simulink model "gm_sla_VHT_HDL1080p_fil_org"  (R2015a)
settings: Solver=FixedStepDiscrete  SolverMode=SingleTasking  StartTime=0.0  StopTime=2200*1125*100  FixedStep=1  RelTol=1e-3
PreLoadFcn:
  | H = fspecial('unsharp')
undefined symbols (not defined in the file): gray
libraries: simulink x6, visionsinks x3, visionhdlio x2, visionhdlconversions x1, visionhdlfilter x1, fillib x1, visionconversions x1, visiongeotforms x1, dspvision x1
settings Model: SimulationMode=accelerator  CovSFcnEnable=off  Creator=yutengz  LastModifiedBy=amatsumo
settings OptimizationCC: BlockReduction=off  BooleanDataType=off  ConditionallyExecuteInputs=off  InlineParams=on
settings DebuggingCC: AlgebraicLoopMsg=error  SaveWithParameterizedLinksMsg=none  UnderspecifiedInitializationDetection=Classic  MergeDetectMultiDrivingBlocksExec=none  SignalResolutionControl=TryResolveAllWithWarning  InheritedTsInSrcMsg=none
settings HardwareCC: ProdHWDeviceType=ASIC/FPGA->ASIC/FPGA  TargetUnknown=on  ProdEqTarget=off

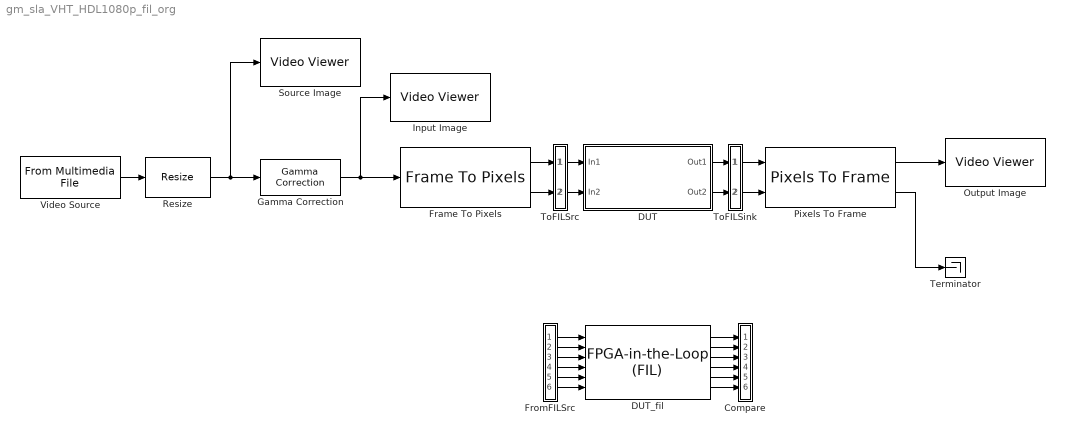
== system gm_sla_VHT_HDL1080p_fil_org ==
  Compare : Subsystem
      mask Display: disp('')
  DUT : Subsystem
  DUT_fil : fillib/FPGA-in-the-Loop (FIL)  ForceInterfaceUpdate=0.90579
  Frame To Pixels : visionhdlio/Frame To Pixels  NumComponents=1  VideoFormat=1080p  ActivePixelsPerLine=32  ActiveVideoLines=18  TotalPixelsPerLine=42  TotalVideoLines=28  StartingActiveLine=6  FrontPorch=5  SampleTime=0
  FromFILSrc : Subsystem
      mask Display: disp('')
  Gamma Correction : visionconversions/Gamma Correction  operation=De-gamma  gamma=2.2  linearSegment=on  breakPoint=0.018
  Input Image : visionsinks/Video Viewer  inputType=Obsolete7b  imagePorts=One multidimensional signal  useColorMap=off  colormapValue=gray(256)  specRange=off  minInputVal=0  maxInputVal=255  FigPos=[366 381 334 275]  AxisZoom=on  trueSizedOnce=off  OpenAtMdlStart=on  DefaultConfigurationName=vipscopes.VideoViewerScopeCfg
  Output Image : visionsinks/Video Viewer  inputType=Obsolete7b  imagePorts=One multidimensional signal  useColorMap=off  colormapValue=gray(256)  specRange=off  minInputVal=0  maxInputVal=255  FigPos=[709 384 334 275]  AxisZoom=on  trueSizedOnce=off  OpenAtMdlStart=on  DefaultConfigurationName=vipscopes.VideoViewerScopeCfg
  Pixels To Frame : visionhdlio/Pixels To Frame  NumComponents=1  VideoFormat=1080p  ActivePixelsPerLine=32  ActiveVideoLines=18  TotalPixelsPerLine=42  TotalVideoLines=28
  Resize : visiongeotforms/Resize  specify=Number of output rows and columns  rfactor=[200 150]  outCols=25  outRows=25  outRowsCols=[1080 1920]  interp_method=Bilinear  antialias=on  useROI=off  roiFlag=off  prodOutputMode=Binary point scaling  prodOutputWordLength=32  prodOutputFracLength=10  roundingMode=Nearest  overflowMode=on
  Source Image : visionsinks/Video Viewer  inputType=Obsolete7b  imagePorts=One multidimensional signal  useColorMap=off  colormapValue=gray(256)  specRange=off  minInputVal=0  maxInputVal=255  FigPos=[21 379 334 275]  AxisZoom=on  trueSizedOnce=off  OpenAtMdlStart=on  DefaultConfigurationName=vipscopes.VideoViewerScopeCfg
  Terminator : Terminator
  ToFILSink : Subsystem
      mask Display: disp('')
  ToFILSrc : Subsystem
      mask Display: disp('')
  Video Source : dspvision/From Multimedia File  inputFilename=rhinos.avi  loop=on  numPlays=inf  outputStreams=Video only  videoDataType=uint8  audioDataType=int16  inheritSampleTime=off  userDefinedSampleTime="1125*2200  %402*324"  noAudioOutput=off  isIntensityVideo=off  fourcc=Intensity  colorVideoFormat=One multidimensional signal  outputEOF=off  dataOrg=Column-major  audioFrameSize=1024  computeAudioFrameSize=off  outSamplingMode=Sample based
  wires:
  Video Source/1 -> Resize/1
  Pixels To Frame/1 -> Output Image/1
  Pixels To Frame/2 -> Terminator/1
  Gamma Correction/1 -> Input Image/1, Frame To Pixels/1
  Resize/1 -> Source Image/1, Gamma Correction/1
  ToFILSrc/1(out1) -> DUT/1(In1)
  ToFILSrc/2(out2) -> DUT/2(In2)
  DUT/1(Out1) -> ToFILSink/1(in1)
  DUT/2(Out2) -> ToFILSink/2(in2)
  Frame To Pixels/1 -> ToFILSrc/1(in1)
  Frame To Pixels/2 -> ToFILSrc/2(in2)
  ToFILSink/1(out1) -> Pixels To Frame/1
  ToFILSink/2(out2) -> Pixels To Frame/2
  FromFILSrc/1(out1) -> DUT_fil/1
  FromFILSrc/2(out2) -> DUT_fil/2
  FromFILSrc/3(out3) -> DUT_fil/3
  FromFILSrc/4(out4) -> DUT_fil/4
  FromFILSrc/5(out5) -> DUT_fil/5
  FromFILSrc/6(out6) -> DUT_fil/6
  DUT_fil/1 -> Compare/1(in1)
  DUT_fil/2 -> Compare/2(in2)
  DUT_fil/3 -> Compare/3(in3)
  DUT_fil/4 -> Compare/4(in4)
  DUT_fil/5 -> Compare/5(in5)
  DUT_fil/6 -> Compare/6(in6)

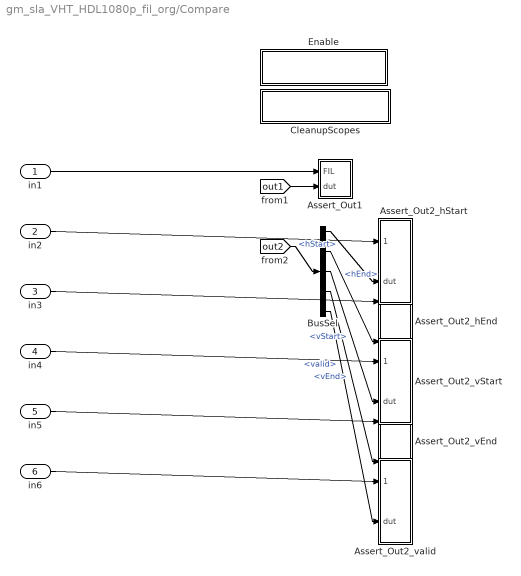
== system gm_sla_VHT_HDL1080p_fil_org/Compare ==
  in1 : Inport
  in2 : Inport  Port=2
  in3 : Inport  Port=3
  in4 : Inport  Port=4
  in5 : Inport  Port=5
  in6 : Inport  Port=6
  Assert_Out1 : Subsystem
  Assert_Out2_hEnd : Subsystem
  Assert_Out2_hStart : Subsystem
  Assert_Out2_vEnd : Subsystem
  Assert_Out2_vStart : Subsystem
  Assert_Out2_valid : Subsystem
  BusSel : BusSelector  OutputSignals=hStart,hEnd,vStart,vEnd,valid
  CleanupScopes : Subsystem
      settings: OpenFcn=|
      | blkName = gcb;
      | idx = regexp(blkName, '/CleanupScopes$', 'once');
      | blkParent = blkName(1:idx-1);
      | blks=find_system(blkParent, 'blocktype', 'Scope');
      | e = get_param(blks{1}, 'Open');
      | if strcmp(e, 'on'), f= 'off'; else f = 'on'; end
      | for ii=1:length(blks), set_param(blks{ii}, 'Open', f); end; drawnow;
      mask Display: disp(['Double click to\n turn on/off all scopes'])
  Enable : Subsystem
      settings: OpenFcn=|
      | blkName = gcb;
      | idx = regexp(blkName, '/Enable$', 'once');
      | blkParent = blkName(1:idx-1);
      | blks=find_system(blkParent, 'blocktype', 'Assertion');
      | e = get_param(blks{1}, 'Enabled');
      | if strcmp(e, 'on'), f= 'off';, else, f = 'on';, end
      | for ii=1:length(blks), set_param(blks{ii}, 'Enabled', f);, end
      | dispMsg = sprintf('disp([''Double click to turn %s \\n all Assertions''])', upper(e));
      | set_param(gcb, 'MaskDisplay', dispMsg);
      mask Display: disp(['Double click to turn OFF \n all Assertions'])
  wires:
  [out2] -> BusSel/1
  in1/1 -> Assert_Out1/1(FIL)
  [out1] -> Assert_Out1/2(dut)
  in2/1 -> Assert_Out2_hStart/1(cosim)
  BusSel/1 -> Assert_Out2_hStart/2(dut)  "<hStart>"
  in3/1 -> Assert_Out2_hEnd/1(cosim)
  BusSel/2 -> Assert_Out2_hEnd/2(dut)  "<hEnd>"
  in4/1 -> Assert_Out2_vStart/1(cosim)
  BusSel/3 -> Assert_Out2_vStart/2(dut)  "<vStart>"
  in5/1 -> Assert_Out2_vEnd/1(cosim)
  BusSel/4 -> Assert_Out2_vEnd/2(dut)  "<vEnd>"
  in6/1 -> Assert_Out2_valid/1(cosim)
  BusSel/5 -> Assert_Out2_valid/2(dut)  "<valid>"

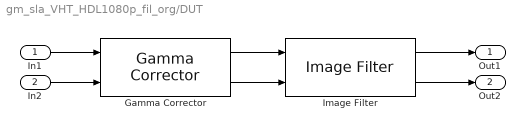
== system gm_sla_VHT_HDL1080p_fil_org/DUT ==
  In1 : Inport
  In2 : Inport  Port=2
  Gamma Corrector : visionhdlconversions/Gamma Corrector  Correction=Gamma  Gamma=2.2  LinearSegment=on  BreakPoint=0.018  SimulateUsing=Code generation
  Image Filter : visionhdlfilter/Image Filter  Coefficients=H  PaddingMethod=Replicate  PaddingValue=0  LineBufferSize=2048  roundingMode=Floor  overflowMode=on  CoeffDataTypeStr=fixdt(1,8,4)  CoeffMin=[]  CoeffMax=[]  OutputMin=[]  OutputMax=[]  SimulateUsing=Code generation
  Out1 : Outport
  Out2 : Outport  Port=2
  wires:
  In2/1 -> Gamma Corrector/2
  Gamma Corrector/2 -> Image Filter/2
  In1/1 -> Gamma Corrector/1
  Image Filter/2 -> Out2/1
  Gamma Corrector/1 -> Image Filter/1
  Image Filter/1 -> Out1/1

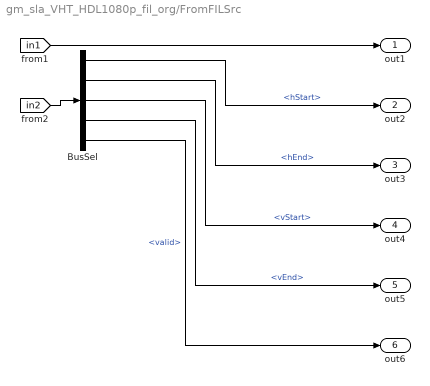
== system gm_sla_VHT_HDL1080p_fil_org/FromFILSrc ==
  BusSel : BusSelector  OutputSignals=hStart,hEnd,vStart,vEnd,valid
  out1 : Outport
  out2 : Outport  Port=2
  out3 : Outport  Port=3
  out4 : Outport  Port=4
  out5 : Outport  Port=5
  out6 : Outport  Port=6
  wires:
  [in2] -> BusSel/1
  [in1] -> out1/1
  BusSel/1 -> out2/1  "<hStart>"
  BusSel/2 -> out3/1  "<hEnd>"
  BusSel/3 -> out4/1  "<vStart>"
  BusSel/4 -> out5/1  "<vEnd>"
  BusSel/5 -> out6/1  "<valid>"

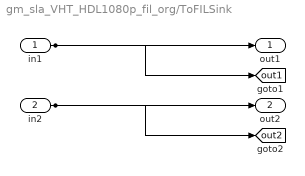
== system gm_sla_VHT_HDL1080p_fil_org/ToFILSink ==
  in1 : Inport
  in2 : Inport  Port=2
  out1 : Outport
  out2 : Outport  Port=2
  tag scope: out1=global, out2=global
  wires:
  in1/1 -> out1/1, [out1]
  in2/1 -> out2/1, [out2]

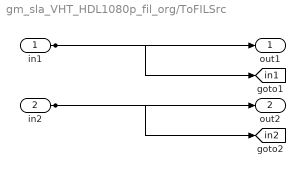
== system gm_sla_VHT_HDL1080p_fil_org/ToFILSrc ==
  in1 : Inport
  in2 : Inport  Port=2
  out1 : Outport
  out2 : Outport  Port=2
  tag scope: in1=global, in2=global
  wires:
  in1/1 -> out1/1, [in1]
  in2/1 -> out2/1, [in2]

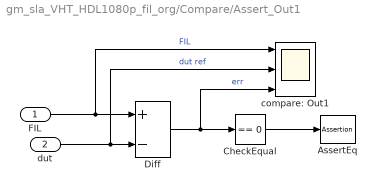
== system gm_sla_VHT_HDL1080p_fil_org/Compare/Assert_Out1 ==
  FIL : Inport
  dut : Inport  Port=2
  AssertEq : Assertion  StopWhenAssertionFail=off
  CheckEqual : simulink/Logic and Bit Operations/Compare To Zero  relop===  OutDataTypeStr=uint8  ZeroCross=off
  Diff : Sum  Inputs=+-
  compare: Out1 : Scope  NumInputPorts=3
      settings: YMin=-5~-5~-5  YMax=5~5~5
  wires:
  CheckEqual/1 -> AssertEq/1
  dut/1 -> Diff/2, compare: Out1/2  "dut ref"
  FIL/1 -> compare: Out1/1, Diff/1  "FIL"
  Diff/1 -> CheckEqual/1, compare: Out1/3  "err"

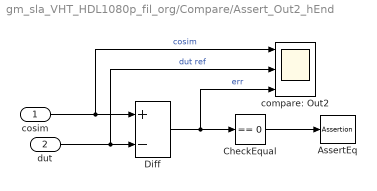
== system gm_sla_VHT_HDL1080p_fil_org/Compare/Assert_Out2_hEnd ==
  cosim : Inport
  dut : Inport  Port=2
  AssertEq : Assertion  StopWhenAssertionFail=off
  CheckEqual : simulink/Logic and Bit Operations/Compare To Zero  relop===  OutDataTypeStr=uint8  ZeroCross=off
  Diff : Sum  Inputs=+-
  compare: Out2 : Scope  NumInputPorts=3
      settings: YMin=-5~-5~-5  YMax=5~5~5
  wires:
  CheckEqual/1 -> AssertEq/1
  dut/1 -> Diff/2, compare: Out2/2  "dut ref"
  cosim/1 -> compare: Out2/1, Diff/1  "cosim"
  Diff/1 -> CheckEqual/1, compare: Out2/3  "err"

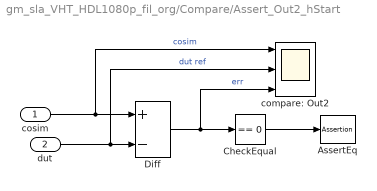
== system gm_sla_VHT_HDL1080p_fil_org/Compare/Assert_Out2_hStart ==
  cosim : Inport
  dut : Inport  Port=2
  AssertEq : Assertion  StopWhenAssertionFail=off
  CheckEqual : simulink/Logic and Bit Operations/Compare To Zero  relop===  OutDataTypeStr=uint8  ZeroCross=off
  Diff : Sum  Inputs=+-
  compare: Out2 : Scope  NumInputPorts=3
      settings: YMin=-5~-5~-5  YMax=5~5~5
  wires:
  CheckEqual/1 -> AssertEq/1
  dut/1 -> Diff/2, compare: Out2/2  "dut ref"
  cosim/1 -> compare: Out2/1, Diff/1  "cosim"
  Diff/1 -> CheckEqual/1, compare: Out2/3  "err"

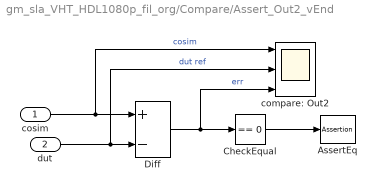
== system gm_sla_VHT_HDL1080p_fil_org/Compare/Assert_Out2_vEnd ==
  cosim : Inport
  dut : Inport  Port=2
  AssertEq : Assertion  StopWhenAssertionFail=off
  CheckEqual : simulink/Logic and Bit Operations/Compare To Zero  relop===  OutDataTypeStr=uint8  ZeroCross=off
  Diff : Sum  Inputs=+-
  compare: Out2 : Scope  NumInputPorts=3
      settings: YMin=-5~-5~-5  YMax=5~5~5
  wires:
  CheckEqual/1 -> AssertEq/1
  dut/1 -> Diff/2, compare: Out2/2  "dut ref"
  cosim/1 -> compare: Out2/1, Diff/1  "cosim"
  Diff/1 -> CheckEqual/1, compare: Out2/3  "err"

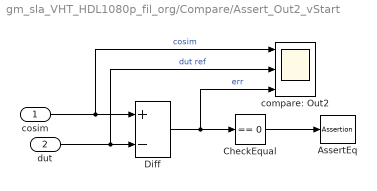
== system gm_sla_VHT_HDL1080p_fil_org/Compare/Assert_Out2_vStart ==
  cosim : Inport
  dut : Inport  Port=2
  AssertEq : Assertion  StopWhenAssertionFail=off
  CheckEqual : simulink/Logic and Bit Operations/Compare To Zero  relop===  OutDataTypeStr=uint8  ZeroCross=off
  Diff : Sum  Inputs=+-
  compare: Out2 : Scope  NumInputPorts=3
      settings: YMin=-5~-5~-5  YMax=5~5~5
  wires:
  CheckEqual/1 -> AssertEq/1
  dut/1 -> Diff/2, compare: Out2/2  "dut ref"
  cosim/1 -> compare: Out2/1, Diff/1  "cosim"
  Diff/1 -> CheckEqual/1, compare: Out2/3  "err"

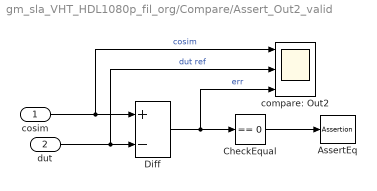
== system gm_sla_VHT_HDL1080p_fil_org/Compare/Assert_Out2_valid ==
  cosim : Inport
  dut : Inport  Port=2
  AssertEq : Assertion  StopWhenAssertionFail=off
  CheckEqual : simulink/Logic and Bit Operations/Compare To Zero  relop===  OutDataTypeStr=uint8  ZeroCross=off
  Diff : Sum  Inputs=+-
  compare: Out2 : Scope  NumInputPorts=3
      settings: YMin=-5~-5~-5  YMax=5~5~5
  wires:
  CheckEqual/1 -> AssertEq/1
  dut/1 -> Diff/2, compare: Out2/2  "dut ref"
  cosim/1 -> compare: Out2/1, Diff/1  "cosim"
  Diff/1 -> CheckEqual/1, compare: Out2/3  "err"

== system gm_sla_VHT_HDL1080p_fil_org/Compare/CleanupScopes ==

== system gm_sla_VHT_HDL1080p_fil_org/Compare/Enable ==
